simulink model "deteccion_aislamiento_falla"  (R2018a)
settings: Solver=VariableStepAuto  StartTime=0.0  StopTime=.5  FixedStep=1e-6  MaxStep=1e-4  RelTol=1e-3
PreLoadFcn:
  | SimulinkInit
InitFcn:
  | SimulinkInit
StopFcn:
  | EndingScript
undefined symbols (not defined in the file or in its folder): f, ssAl, ssBl, ssCl
libraries: instrumentlib x8
settings Model: Creator=erich  LastModifiedBy=MarioAndres
settings CodeAppCC: StateflowObjectComments=on
settings SimscapeCC: SimscapeNormalizeSystem=off

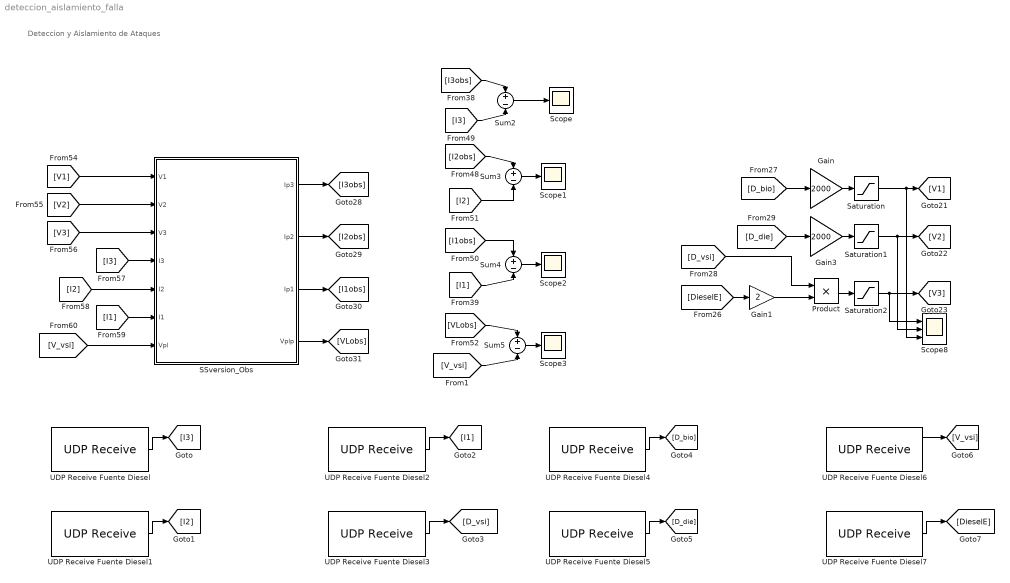
== system deteccion_aislamiento_falla ==
  note: Deteccion y Aislamiento de Ataques
  Gain : Gain  Gain=2000
  Gain1 : Gain  Gain=2
  Gain3 : Gain  Gain=2000
  Product : Product
  SSversion_Obs : Subsystem
  Saturation : Saturate  UpperLimit=1000  LowerLimit=-1000
  Saturation1 : Saturate  UpperLimit=1000  LowerLimit=-1000
  Saturation2 : Saturate  UpperLimit=1000  LowerLimit=-1000
  Scope{,1..3} (4 alike) : Scope
  Scope8 : Scope  NumInputPorts=3
  Sum{2..5} (4 alike) : Sum  Inputs=+-
  UDP Receive Fuente Diesel : instrumentlib/UDP Receive  Host=172.16.49.88  Port=8887  LocalPort=8886  EnablePortSharing=off  GetLatestData=off  DataSize=1  DataType=double  ASCIIFormatting=%f,  Terminator=LF  ByteOrder=BigEndian  EnableBlockingMode=on  Timeout=100  SampleTime=-1  LocalAddress=0.0.0.0
      settings: SourceProductName=Instrument Control Toolbox
  UDP Receive Fuente Diesel1 : instrumentlib/UDP Receive  Host=172.16.49.83  Port=8887  LocalPort=8886  EnablePortSharing=off  GetLatestData=off  DataSize=1  DataType=double  ASCIIFormatting=%f,  Terminator=LF  ByteOrder=BigEndian  EnableBlockingMode=on  Timeout=100  SampleTime=-1  LocalAddress=0.0.0.0
      settings: SourceProductName=Instrument Control Toolbox
  UDP Receive Fuente Diesel2 : instrumentlib/UDP Receive  Host=172.16.49.102  Port=8887  LocalPort=8886  EnablePortSharing=off  GetLatestData=off  DataSize=1  DataType=double  ASCIIFormatting=%f,  Terminator=LF  ByteOrder=BigEndian  EnableBlockingMode=on  Timeout=100  SampleTime=-1  LocalAddress=0.0.0.0
      settings: SourceProductName=Instrument Control Toolbox
  UDP Receive Fuente Diesel3 : instrumentlib/UDP Receive  Host=172.16.49.88  Port=8887  LocalPort=8885  EnablePortSharing=off  GetLatestData=off  DataSize=1  DataType=double  ASCIIFormatting=%f,  Terminator=LF  ByteOrder=BigEndian  EnableBlockingMode=on  Timeout=100  SampleTime=-1  LocalAddress=0.0.0.0
      settings: SourceProductName=Instrument Control Toolbox
  UDP Receive Fuente Diesel4 : instrumentlib/UDP Receive  Host=172.16.49.102  Port=8887  LocalPort=8885  EnablePortSharing=off  GetLatestData=off  DataSize=1  DataType=double  ASCIIFormatting=%f,  Terminator=LF  ByteOrder=BigEndian  EnableBlockingMode=on  Timeout=100  SampleTime=-1  LocalAddress=0.0.0.0
      settings: SourceProductName=Instrument Control Toolbox
  UDP Receive Fuente Diesel5 : instrumentlib/UDP Receive  Host=172.16.49.83  Port=8887  LocalPort=8885  EnablePortSharing=off  GetLatestData=off  DataSize=1  DataType=double  ASCIIFormatting=%f,  Terminator=LF  ByteOrder=BigEndian  EnableBlockingMode=on  Timeout=100  SampleTime=-1  LocalAddress=0.0.0.0
      settings: SourceProductName=Instrument Control Toolbox
  UDP Receive Fuente Diesel6 : instrumentlib/UDP Receive  Host=172.16.49.104  Port=8887  LocalPort=8886  EnablePortSharing=off  GetLatestData=off  DataSize=1  DataType=double  ASCIIFormatting=%f,  Terminator=LF  ByteOrder=BigEndian  EnableBlockingMode=off  Timeout=100  SampleTime=-1  LocalAddress=0.0.0.0
      settings: SourceProductName=Instrument Control Toolbox
  UDP Receive Fuente Diesel7 : instrumentlib/UDP Receive  Host=172.16.49.88  Port=8887  LocalPort=8884  EnablePortSharing=off  GetLatestData=off  DataSize=1  DataType=double  ASCIIFormatting=%f,  Terminator=LF  ByteOrder=BigEndian  EnableBlockingMode=on  Timeout=100  SampleTime=-1  LocalAddress=0.0.0.0
      settings: SourceProductName=Instrument Control Toolbox
  wires:
  [D_bio] -> Gain/1
  Gain/1 -> Saturation/1
  Saturation/1 -> [V1], Scope8/3
  Saturation1/1 -> Scope8/2, [V2]
  Saturation2/1 -> [V3], Scope8/1
  Product/1 -> Saturation2/1
  Sum2/1 -> Scope/1
  [I3] -> Sum2/2
  Sum4/1 -> Scope2/1
  [VLobs] -> Sum5/1
  [I2obs] -> Sum3/1
  [I1] -> Sum4/2
  Sum3/1 -> Scope1/1
  [I1obs] -> Sum4/1
  [V_vsi] -> Sum5/2
  Sum5/1 -> Scope3/1
  [I2] -> Sum3/2
  [I3obs] -> Sum2/1
  [D_vsi] -> Product/1
  [V1] -> SSversion_Obs/1(V1)
  [V2] -> SSversion_Obs/2(V2)
  [V3] -> SSversion_Obs/3(V3)
  [I3] -> SSversion_Obs/4(I3)
  [I2] -> SSversion_Obs/5(I2)
  [I1] -> SSversion_Obs/6(I1)
  [V_vsi] -> SSversion_Obs/7(Vpl)
  SSversion_Obs/1(Ip3) -> [I3obs]
  SSversion_Obs/2(Ip2) -> [I2obs]
  SSversion_Obs/3(Ip1) -> [I1obs]
  SSversion_Obs/4(Vplp) -> [VLobs]
  [DieselE] -> Gain1/1
  Gain3/1 -> Saturation1/1
  [D_die] -> Gain3/1
  Gain1/1 -> Product/2
  UDP Receive Fuente Diesel/1 -> [I3]
  UDP Receive Fuente Diesel1/1 -> [I2]
  UDP Receive Fuente Diesel2/1 -> [I1]
  UDP Receive Fuente Diesel3/1 -> [D_vsi]
  UDP Receive Fuente Diesel6/1 -> [V_vsi]
  UDP Receive Fuente Diesel7/1 -> [DieselE]
  UDP Receive Fuente Diesel5/1 -> [D_die]
  UDP Receive Fuente Diesel4/1 -> [D_bio]

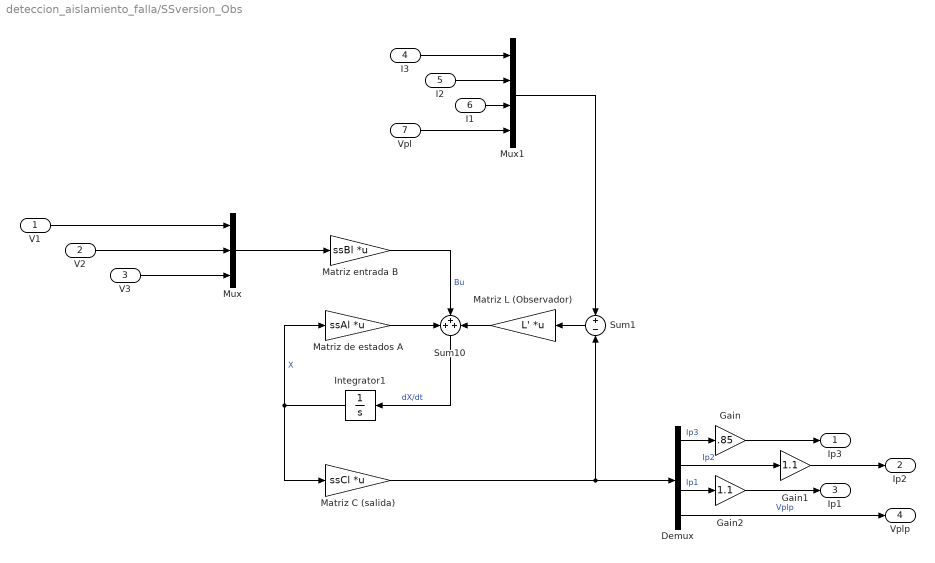
== system deteccion_aislamiento_falla/SSversion_Obs ==
  V1 : Inport
  V2 : Inport  Port=2
  V3 : Inport  Port=3
  I3 : Inport  Port=4
  I2 : Inport  Port=5
  I1 : Inport  Port=6
  Vpl : Inport  Port=7
  Demux : Demux
  Gain : Gain  Gain=.85
  Gain1 : Gain  Gain=1.1
  Gain2 : Gain  Gain=1.1
  Integrator1 : Integrator
  Matriz C (salida) : Gain  Gain=ssCl  Multiplication=Matrix(K*u)
  Matriz L (Observador) : Gain  Gain=L'  Multiplication=Matrix(K*u)
  Matriz de estados A : Gain  Gain=ssAl  Multiplication=Matrix(K*u)
  Matriz entrada B : Gain  Gain=ssBl  Multiplication=Matrix(K*u)
  Mux : Mux  Inputs=3
  Mux1 : Mux
  Sum1 : Sum  Inputs=+|-
  Sum10 : Sum  Inputs=+++
  Ip3 : Outport
  Ip2 : Outport  Port=2
  Ip1 : Outport  Port=3
  Vplp : Outport  Port=4
  wires:
  Matriz C (salida)/1 -> Demux/1, Sum1/2
  V1/1 -> Mux/1
  V2/1 -> Mux/2
  Demux/3 -> Gain2/1  "Ip1"
  V3/1 -> Mux/3
  Mux/1 -> Matriz entrada B/1
  Sum10/1 -> Integrator1/1  "dX/dt"
  Demux/2 -> Gain1/1  "Ip2"
  Demux/4 -> Vplp/1  "Vplp"
  Integrator1/1 -> Matriz de estados A/1, Matriz C (salida)/1  "X"
  Demux/1 -> Gain/1  "Ip3"
  Matriz de estados A/1 -> Sum10/1
  Matriz entrada B/1 -> Sum10/2  "Bu"
  I2/1 -> Mux1/2
  I3/1 -> Mux1/1
  I1/1 -> Mux1/3
  Vpl/1 -> Mux1/4
  Matriz L (Observador)/1 -> Sum10/3
  Sum1/1 -> Matriz L (Observador)/1
  Mux1/1 -> Sum1/1
  Gain/1 -> Ip3/1
  Gain1/1 -> Ip2/1
  Gain2/1 -> Ip1/1
